simulink model "motor_supervisor"  (R2023b)
settings: Solver=FixedStepDiscrete  StartTime=0.0  StopTime=10.0  FixedStep=1e-3  RelTol=1e-3  EnableMultiTasking=on
settings Model: DataDictionary=common.sldd  Creator=mfussi  LastModifiedBy=mfussi
settings SolverCC: AutoInsertRateTranBlk=on  InsertRTBMode=Never (minimum delay)
settings DataIOCC: SaveOutput=off  SignalLogging=off  DSMLogging=off  StreamToWks=off  SaveTime=off  ReturnWorkspaceOutputs=off
settings OptimizationCC: DefaultParameterBehavior=Inlined  UseDivisionForNetSlopeComputation=on  GainParamInheritBuiltInType=on  UseFloatMulNetSlope=on  InlineInvariantSignals=on  EnhancedBackFolding=on  NoFixptDivByZeroProtection=on  EfficientFloat2IntCast=on  OptimizeBlockOrder=speed  DifferentSizesBufferReuse=on  OptimizationCustomize=off  EfficientTunableParamExpr=on
settings DebuggingCC: ParameterTunabilityLossMsg=error
settings HardwareCC: ProdBitPerPointer=32  ProdBitPerSizeT=32  ProdBitPerPtrDiffT=32  ProdLargestAtomicInteger=Long  ProdLargestAtomicFloat=Double  ProdWordSize=32  ProdLongLongMode=on  ProdHWDeviceType=ARM Compatible->ARM Cortex-M
settings SFSimCC: MATLABDynamicMemAlloc=off
settings SFSimCC: SimCustomHeaderCode=|
  | #include "rtw_enable_disable_motors.h"
  | #include "rtw_motor_config.h"
settings SFSimCC: SimUserSources=|
  | rtw_enable_disable_motors.c
  | rtw_motor_config.c
settings RTWCC: Description=Embedded Coder  SystemTargetFile=ert.tlc  GenCodeOnly=on  TemplateMakefile=ert_default_tmf  RTWUseSimCustomCode=on
settings RTWCC: CustomHeaderCode=|
  | #include "rtw_enable_disable_motors.h"
  | #include "rtw_motor_config.h"
settings RTWCC: CustomSource=|
  | rtw_enable_disable_motors.c
  | rtw_motor_config.c
settings CodeAppCC: ForceParamTrailComments=on  IgnoreCustomStorageClasses=off  OperatorAnnotations=on  SimulinkDataObjDesc=on  SFDataObjDesc=on  InsertBlockDesc=on
settings ERTTargetCC: TargetLangStandard=C99 (ISO)  CodeReplacementLibrary=ARM Cortex-M,iCubTech  GenerateSampleERTMain=on  CodeInterfacePackaging=Reusable function  InlinedParameterPlacement=NonHierarchical  RootIOFormat=Structure reference  ERTCustomFileTemplate=example_file_process.tlc

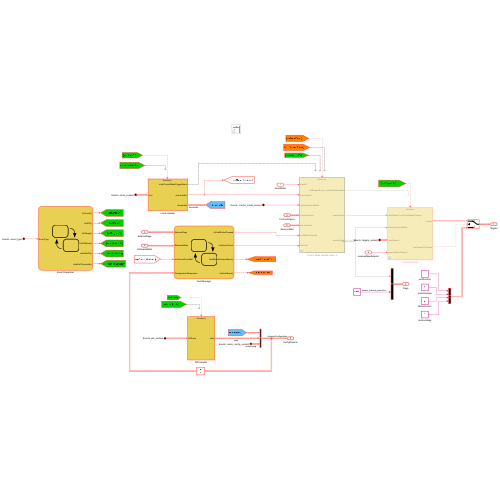
[thumbnail: Simulink's stored preview of the top-level diagram]
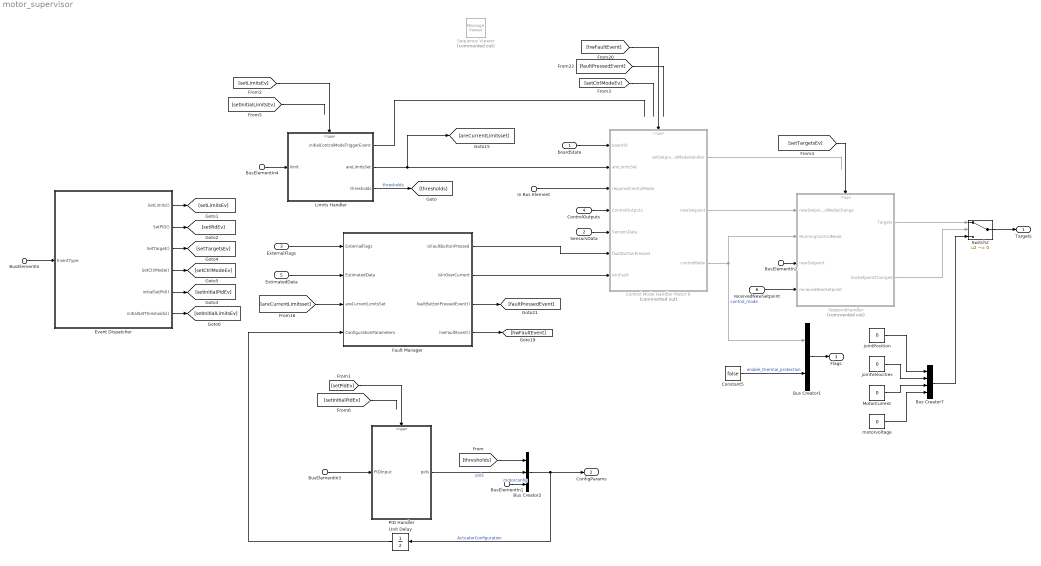
== system motor_supervisor ==
  boardState : Inport
  SensorsData : Inport  Port=2  OutDataTypeStr=Bus: SensorsData  BusOutputAsStruct=on
  ExternalFlags : Inport  Port=3  OutDataTypeStr=Bus: ExternalFlags  BusOutputAsStruct=on
  ControlOutputs : Inport  Port=4  OutDataTypeStr=Bus: FOCOutputs  BusOutputAsStruct=on
  EstimatedData : Inport  Port=5  OutDataTypeStr=Bus: EstimatedData  BusOutputAsStruct=on
  receivedNewSetpoint : Inport  Port=6
  BusElementIn2 : Inport  Port=7  PortName=Events  Element=targets_content
  BusElementIn3 : Inport  Port=7  PortName=Events  Element=pid_content
  In Bus Element : Inport  Port=7  PortName=Events  Element=control_mode_content
  BusElementIn4 : Inport  Port=7  PortName=Events  Element=limits_content
  BusElementIn : Inport  Port=7  PortName=Events  Element=event_type
  BusElementIn1 : Inport  Port=7  PortName=Events  Element=motor_config_content
  Bus Creator1 : BusCreator  Inputs=2  OutDataTypeStr=Bus: Flags  NonVirtualBus=on
      settings: InheritFromInputs=off
  Bus Creator2 : BusCreator  Inputs=3  OutDataTypeStr=Bus: ActuatorConfiguration  NonVirtualBus=on
      settings: InheritFromInputs=off
  Bus Creator7 : BusCreator  Inputs=4  OutDataTypeStr=Bus: Targets  NonVirtualBus=on
      settings: InheritFromInputs=off
  Constant5 : Constant  Value=false  OutDataTypeStr=boolean
  Control Mode Handler Motor 0 : Subsystem  Commented=on  TreatAsAtomicUnit=on
  Event Dispatcher : Stateflow chart  TreatAsAtomicUnit=on
  Fault Manager : Stateflow chart  TreatAsAtomicUnit=on
  Limits Handler : Subsystem  TreatAsAtomicUnit=on
  MotorCurrent : Constant  Value=0  OutDataTypeStr=single
  PID Handler : Subsystem
  Sequence Viewer : MessageViewer  Commented=on  History=1000  SavedRootId=#
  SetpointHandler : Subsystem  Commented=on  TreatAsAtomicUnit=on
  Switch2 : Switch  Criteria=u2 ~= 0  OutDataTypeStr=Inherit: Inherit via back propagation  SaturateOnIntegerOverflow=off  InputSameDT=off
  Unit Delay : UnitDelay  SampleTime=-1  HasFrameUpgradeWarning=on
  jointPosition : Constant  Value=0  OutDataTypeStr=single
  jointVelocities : Constant  Value=0  OutDataTypeStr=single
  motorvoltage : Constant  Value=0  OutDataTypeStr=single
  Targets : Outport  OutDataTypeStr=Bus: Targets
  ConfigParams : Outport  Port=2  OutDataTypeStr=Bus: ActuatorConfiguration
  Flags : Outport  Port=3  OutDataTypeStr=Bus: Flags
  wires:
  Switch2/1 -> Targets/1
  ControlOutputs/1 -> Control Mode Handler Motor 0/4(ControlOutputs)
  boardState/1 -> Control Mode Handler Motor 0/1(boardSt)
  ExternalFlags/1 -> Fault Manager/1(ExternalFlags)
  [setLimitsEv] -> Limits Handler/Trigger
  EstimatedData/1 -> Fault Manager/2(EstimatedData)
  [faultPressedEvent] -> ?
  Fault Manager/1(isFaultButtonPressed) -> Control Mode Handler Motor 0/6(faultButtonPressed)
  SensorsData/1 -> Control Mode Handler Motor 0/5(SensorsData)
  [setPidEv] -> PID Handler/Trigger
  Fault Manager/4(hwFaultEvent()) -> [hwFaultEvent]
  Bus Creator2/1 -> ConfigParams/1, Unit Delay/1  "ActuatorConfiguration"
  Control Mode Handler Motor 0/1(setSetpointEvent_controlModeHandler) -> ?
  Unit Delay/1 -> Fault Manager/4(ConfigurationParameters)
  MotorCurrent/1 -> Bus Creator7/3
  Fault Manager/2(isInOverCurrent) -> Control Mode Handler Motor 0/7(isInFault)
  SetpointHandler/2(hasSetpointChanged) -> Switch2/2
  In Bus Element/1 -> Control Mode Handler Motor 0/3(requiredControlMode)
  [hwFaultEvent] -> Control Mode Handler Motor 0/Trigger
  BusElementIn2/1 -> SetpointHandler/3(newSetpoint)
  BusElementIn1/1 -> Bus Creator2/3  "motorconfig"
  jointPosition/1 -> Bus Creator7/1
  [setInitialLimitsEv] -> ?
  motorvoltage/1 -> Bus Creator7/4
  SetpointHandler/1(Targets) -> Switch2/1
  BusElementIn3/1 -> PID Handler/1(PIDInput)
  [setCtrlModeEv] -> ?
  [setInitialPidEv] -> ?
  Limits Handler/2(areLimitsSet) -> Control Mode Handler Motor 0/2(areLimitsSet), [areCurrentLimitsset]
  [areCurrentLimitsset] -> Fault Manager/3(areCurrentLimitsSet)
  [thresholds] -> Bus Creator2/1
  Fault Manager/3(faultButtonPressedEvent()) -> [faultPressedEvent]
  Limits Handler/1(initialControlModeTriggerEvent) -> ?
  Limits Handler/3(thresholds) -> [thresholds]  "thresholds"
  jointVelocities/1 -> Bus Creator7/2
  Bus Creator7/1 -> Switch2/3
  BusElementIn/1 -> Event Dispatcher/1(EventType)
  Event Dispatcher/1(SetLimits()) -> [setLimitsEv]
  Event Dispatcher/2(SetPID()) -> [setPidEv]
  Event Dispatcher/3(SetTarget()) -> [setTargetsEv]
  Event Dispatcher/4(SetCtrlMode()) -> [setCtrlModeEv]
  Event Dispatcher/5(initialSetPid()) -> [setInitialPidEv]
  Event Dispatcher/6(initialSetThresholds()) -> [setInitialLimitsEv]
  Constant5/1 -> Bus Creator1/2  "enable_thermal_protection"
  Control Mode Handler Motor 0/3(controlMode) -> SetpointHandler/2(RunningControlMode), Bus Creator1/1  "control_mode"
  Bus Creator1/1 -> Flags/1
  Control Mode Handler Motor 0/2(newSetpoint) -> SetpointHandler/1(newSetpoint_onControlModeChange)
  [setTargetsEv] -> SetpointHandler/Trigger
  receivedNewSetpoint/1 -> SetpointHandler/4(receivedNewSetpoint)
  BusElementIn4/1 -> Limits Handler/1(limit)
  PID Handler/1(pids) -> Bus Creator2/2  "pids"

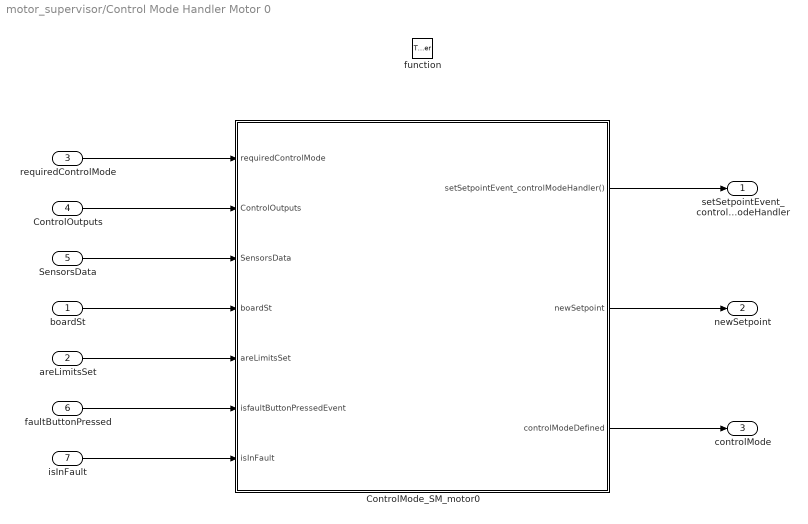
== system motor_supervisor/Control Mode Handler Motor 0 ==
  boardSt : Inport
  areLimitsSet : Inport  Port=2
  requiredControlMode : Inport  Port=3  OutDataTypeStr=Enum: ControlModes
  ControlOutputs : Inport  Port=4  OutDataTypeStr=Bus: FOCOutputs
  SensorsData : Inport  Port=5  OutDataTypeStr=Bus: SensorsData
  faultButtonPressed : Inport  Port=6  OutDataTypeStr=boolean
  isInFault : Inport  Port=7
  function : TriggerPort  TriggerType=function-call  VariantControl=(inherit)  OutputDataType=double
  ControlMode_SM_motor0 : Stateflow chart  TreatAsAtomicUnit=on
      settings: PortSchema="{\"entries\":[{\"content\":{\"sides\":[{\"content\":{\"connectorIds\":[\"In3\",\"In5\",\"In4\",\"In1\",\"In2\",\"In6\",\"In7\"]},\"type\":\"ConnectorPlacement.EquallySpacedRectSide\",\"uuid\":\"16512c25-bd76-4850-9767-5b856cef53aa\"},{\"content\":{\"connectorIds\":[\"Out3\",\"Out1\",\"Out2\"],\"side\":\"RIGHT\"},\"type\":\"ConnectorPlacement.EquallySpacedRectSide\",\"uuid\":\"18a45251-a2e9-43d4-bd88-b12ad9528921\"},{\"content\":{\"connectorIds\":[],\"side\":\"TOP\"},\"type\":\"ConnectorPlacement.EquallySpacedRectSide\",\"uuid\":\"fd5907c5-7215-4be4-b0f8-eb015da6c502\"}]},\"type\":\"ConnectorPlacement.EquallySpacedConnector\",\"uuid\":\"dd0cc5ef-a33e-40fc-9b84-b3bdf02167fe\"}],\"packageUris\":[\"http://schema.mathworks.com/mf0/Connector/R2020b\"],\"version\":\"1.0\"}"
  setSetpointEvent_controlModeHandler : Outport
  newSetpoint : Outport  Port=2  OutDataTypeStr=single
  controlMode : Outport  Port=3  OutDataTypeStr=Enum: ControlModes
  wires:
  boardSt/1 -> ControlMode_SM_motor0/1(boardSt)
  areLimitsSet/1 -> ControlMode_SM_motor0/2(areLimitsSet)
  requiredControlMode/1 -> ControlMode_SM_motor0/3(requiredControlMode)
  SensorsData/1 -> ControlMode_SM_motor0/4(SensorsData)
  ControlOutputs/1 -> ControlMode_SM_motor0/5(ControlOutputs)
  ControlMode_SM_motor0/2(controlModeDefined) -> controlMode/1
  ControlMode_SM_motor0/1(newSetpoint) -> newSetpoint/1
  ControlMode_SM_motor0/3(setSetpointEvent_controlModeHandler()) -> setSetpointEvent_controlModeHandler/1
  faultButtonPressed/1 -> ControlMode_SM_motor0/6(isfaultButtonPressedEvent)
  isInFault/1 -> ControlMode_SM_motor0/7(isInFault)

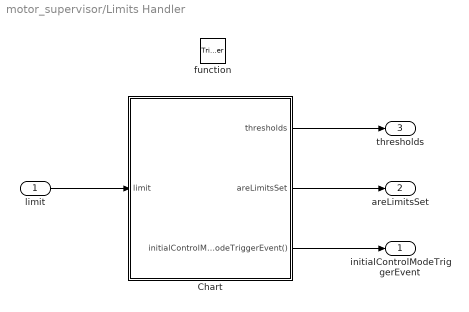
== system motor_supervisor/Limits Handler ==
  limit : Inport  OutDataTypeStr=Bus: SupervisorInputLimits
  function : TriggerPort  TriggerType=function-call  VariantControl=(inherit)
  Chart : Stateflow chart  TreatAsAtomicUnit=on
  initialControlModeTriggerEvent : Outport
  areLimitsSet : Outport  Port=2
  thresholds : Outport  Port=3
  wires:
  Chart/1(thresholds) -> thresholds/1
  Chart/2(areLimitsSet) -> areLimitsSet/1
  limit/1 -> Chart/1(limit)
  Chart/3(initialControlModeTriggerEvent()) -> initialControlModeTriggerEvent/1

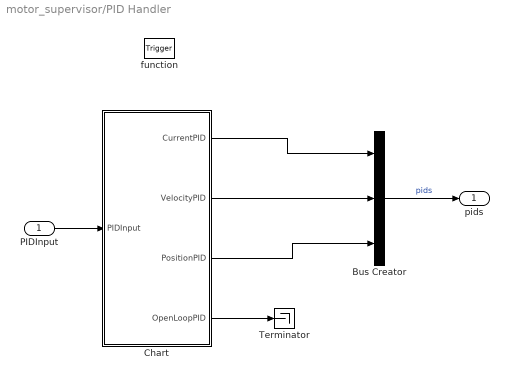
== system motor_supervisor/PID Handler ==
  PIDInput : Inport
  function : TriggerPort  TriggerType=function-call  VariantControl=(inherit)
  Bus Creator : BusCreator  Inputs=3  OutDataTypeStr=Bus: PIDsConfiguration  NonVirtualBus=on
      settings: InheritFromInputs=off
  Chart : Stateflow chart  TreatAsAtomicUnit=on
  Terminator : Terminator
  pids : Outport  OutDataTypeStr=Bus: PIDsConfiguration
  wires:
  PIDInput/1 -> Chart/1(PIDInput)
  Chart/2(VelocityPID) -> Bus Creator/2
  Chart/3(PositionPID) -> Bus Creator/3
  Chart/4(OpenLoopPID) -> Terminator/1
  Chart/1(CurrentPID) -> Bus Creator/1
  Bus Creator/1 -> pids/1  "pids"

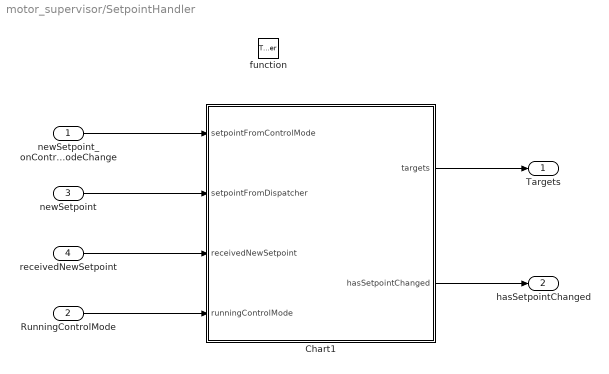
== system motor_supervisor/SetpointHandler ==
  newSetpoint_onControlModeChange : Inport
  RunningControlMode : Inport  Port=2  OutDataTypeStr=Enum: ControlModes
  newSetpoint : Inport  Port=3
  receivedNewSetpoint : Inport  Port=4
  function : TriggerPort  TriggerType=function-call  VariantControl=(inherit)
  Chart1 : Stateflow chart  TreatAsAtomicUnit=on
  Targets : Outport  OutDataTypeStr=Bus: Targets
  hasSetpointChanged : Outport  Port=2
  wires:
  newSetpoint_onControlModeChange/1 -> Chart1/1(setpointFromControlMode)
  newSetpoint/1 -> Chart1/2(setpointFromDispatcher)
  Chart1/2(hasSetpointChanged) -> hasSetpointChanged/1
  Chart1/1(targets) -> Targets/1
  receivedNewSetpoint/1 -> Chart1/3(receivedNewSetpoint)
  RunningControlMode/1 -> Chart1/4(runningControlMode)

== stateflow chart motor_supervisor/Fault Manager ==
  state FAULT_HANDLER
    state OverCurrent [parallel]
      settings: executionOrder=2
      state NoFault
        entry:
        isInOverCurrent=false;
        //MotorFaultFlags.overCurrent=0;
      note: TIP : shall we chage isConfigurationSet,
          | in one function that check only current configuration???
      state LimitNonConfigured
      state OverCurrentFault
        entry:
        //MotorFaultFlags.overCurrent=1;
        isInOverCurrent=true;
        send(hwFaultEvent);
      (default) -> LimitNonConfigured
      LimitNonConfigured -> FAULT_HANDLER.OverCurrent.NoFault : [areCurrentLimitsSet==true]
      FAULT_HANDLER.OverCurrent.NoFault -> OverCurrentFault : [abs(EstimatedData.Iq_filtered) >= ConfigurationParameters.thresholds.motorOverloadCurrents]
      OverCurrentFault -> FAULT_HANDLER.OverCurrent.NoFault : [abs(EstimatedData.Iq_filtered) < ConfigurationParameters.thresholds.motorOverloadCurrents]
    state FaultButtonPressed [parallel]
      settings: executionOrder=1
      state NoFault
        entry:
        isFaultButtonPressed = false;
      state ButtonPressed
        entry:
        isFaultButtonPressed = true;
        send(faultButtonPressedEvent);
      (default) -> FAULT_HANDLER.FaultButtonPressed.NoFault
      ButtonPressed -> FAULT_HANDLER.FaultButtonPressed.NoFault : [hasChangedTo(ExternalFlags.fault_button, false)]
      FAULT_HANDLER.FaultButtonPressed.NoFault -> ButtonPressed : [hasChangedTo(ExternalFlags.fault_button, true)]
  data: isFaultButtonPressed output boolean =false; ExternalFlags input Bus: ExternalFlags; EstimatedData input Bus: EstimatedData; areCurrentLimitsSet input boolean; isInOverCurrent output boolean =false; ConfigurationParameters input Bus: ActuatorConfiguration
  events: faultButtonPressedEvent output FUNCTION_CALL_EVENT; hwFaultEvent output FUNCTION_CALL_EVENT

== stateflow chart motor_supervisor/Event Dispatcher ==
  state Home
  (default) -> (junction 17) : {
      | //Startup Events
      | send(initialSetPid);
      | send(initialSetThresholds)
      | }
  (junction 17) -> Home
  Home -> Home [order 3] : [EventType == SupervisorEvents.SetTarget]{send(SetTarget)}
  Home -> Home [order 1] : [EventType == SupervisorEvents.SetLimit]{send(SetLimits)}
  Home -> Home [order 4] : [EventType == SupervisorEvents.SetControlMode]{send(SetCtrlMode)}
  Home -> Home [order 2] : [EventType == SupervisorEvents.SetPid]{send(SetPID)}
  data: EventType input Enum: SupervisorEvents
  events: SetLimits output FUNCTION_CALL_EVENT; SetPID output FUNCTION_CALL_EVENT; SetTarget output FUNCTION_CALL_EVENT; SetCtrlMode output FUNCTION_CALL_EVENT; initialSetPid output FUNCTION_CALL_EVENT; initialSetThresholds output FUNCTION_CALL_EVENT

== stateflow chart motor_supervisor/PID Handler/Chart ==
  state home
  (default) -> (junction 7)
  (junction 7) -> (junction 9) : {PositionPID = InitConfParams.pids.positionPID;}
  (junction 9) -> (junction 17) [order 5]
  (junction 34) -> (junction 9)
  (junction 9) -> (junction 37) [order 4] : [PIDInput.type == ControlModes.Velocity]
  (junction 9) -> (junction 15) [order 3] : [PIDInput.type == ControlModes.Voltage]
  (junction 9) -> (junction 11) [order 1] : [PIDInput.type == ControlModes.Current]
  (junction 17) -> (junction 27)
  (junction 32) -> (junction 34)
  (junction 9) -> (junction 13) [order 2] : [PIDInput.type == ControlModes.Position]
  (junction 11) -> (junction 19) : {CurrentPID.P = PIDInput.P;
      | CurrentPID.I = PIDInput.I;
      | CurrentPID.D = PIDInput.D;
      | CurrentPID.shift_factor = PIDInput.shift_factor;
      | CurrentPID.type = ControlModes.Current;}
  (junction 13) -> home : {PositionPID.P = 9;
      | PositionPID.I = 15;
      | PositionPID.D = 7;
      | PositionPID.shift_factor = PIDInput.shift_factor;
      | PositionPID.type = ControlModes.Position;}
  (junction 15) -> (junction 24) : {OpenLoopPID.P = PIDInput.P;
      | OpenLoopPID.I = PIDInput.I;
      | OpenLoopPID.D = PIDInput.D;
      | OpenLoopPID.shift_factor = PIDInput.shift_factor;}
  (junction 37) -> (junction 39) : {VelocityPID.P = PIDInput.P;
      | VelocityPID.I = PIDInput.I;
      | VelocityPID.D = PIDInput.D;
      | VelocityPID.shift_factor = PIDInput.shift_factor;}
  (junction 27) -> (junction 39)
  (junction 39) -> (junction 24)
  (junction 19) -> home
  (junction 24) -> home
  home -> (junction 30)
  (junction 30) -> (junction 32)
  data: PIDInput input Bus: PID; CurrentPID output Bus: PID; VelocityPID output Bus: PID; PositionPID output Bus: PID; OpenLoopPID output Bus: PID; InitConfParams local Bus: ActuatorConfiguration

== stateflow chart motor_supervisor/SetpointHandler/Chart1 ==
  note: The idea here is : first of all reset all the targets and then set only the value of the given setpoint. If we are in idel or HW fault all targets remain equal to 0.
  state init
  (junction 54) -> (junction 75) [order 1] : [CheckSetPointVoltage()]{newSetpoint = setpointFromDispatcher.motorvoltage;}
  (junction 75) -> (junction 77)
  (default) -> (junction 8)
  (junction 54) -> (junction 77) [order 2] : [CheckSetPointCurrent()]{newSetpoint = setpointFromDispatcher.motorcurrent;}
  (junction 77) -> (junction 79)
  (junction 8) -> (junction 54) [order 1] : [receivedNewSetpoint==true]
  (junction 9) -> (junction 8)
  (junction 54) -> (junction 79) [order 3] : [CheckSetPointVelocity()]{newSetpoint = setpointFromDispatcher.jointvelocities;}
  (junction 54) -> (junction 81) [order 4] : {newSetpoint = 0;}
  (junction 8) -> (junction 59) [order 2] : {newSetpoint=setpointFromControlMode}
  (junction 22) -> (junction 9)
  (junction 79) -> (junction 81)
  (junction 81) -> (junction 59)
  (junction 59) -> (junction 6) : {targets.motorvoltage = 0;
      | targets.motorcurrent = 0;
      | targets.jointvelocities =0;
      | targets.jointpositions = 0;}
  (junction 6) -> (junction 11) [order 5]
  (junction 6) -> (junction 28) [order 4] : [CheckSetPointPosition()]
  (junction 6) -> (junction 19) [order 2] : [CheckSetPointVoltage()]
  (junction 6) -> (junction 18) [order 3] : [CheckSetPointVelocity()]
  (junction 6) -> (junction 20) [order 1] : [CheckSetPointCurrent()]
  (junction 11) -> (junction 32)
  (junction 18) -> (junction 14) : {targets.jointvelocities = newSetpoint;}
  (junction 28) -> (junction 16) : {targets.jointpositions = newSetpoint;}
  (junction 19) -> (junction 31) : {targets.motorvoltage = newSetpoint;}
  (junction 20) -> (junction 24) : {targets.motorcurrent = newSetpoint;}
  (junction 16) -> (junction 14)
  (junction 14) -> (junction 15)
  (junction 31) -> (junction 24)
  (junction 24) -> (junction 15)
  (junction 15) -> init : {hasSetpointChanged = true;}
  init -> (junction 22)
  (junction 32) -> init
  data: out function_output boolean size=1; out function_output boolean size=1; out function_output boolean size=1; out function_output boolean size=1; setpointFromControlMode input single; setpointFromDispatcher input Bus: Targets; targets output Bus: Targets; hasSetpointChanged output boolean =false; newSetpoint local single size=1; receivedNewSetpoint input boolean; runningControlMode input Enum: ControlModes
  function out = CheckSetPointCurrent:
    | function out = CheckSetPointCurrent
    |  
    | if (runningControlMode ==ControlModes.Current )
    |     out = true;
    | else 
    |     out = false;
    | end
  function out = CheckSetPointVoltage:
    | function out = CheckSetPointVoltage
    |  
    | if (runningControlMode ==ControlModes.Voltage )
    |     out = true;
    | else 
    |     out = false;
    | end
  function out = CheckSetPointPosition:
    | function out = CheckSetPointPosition
    |  
    | if (runningControlMode ==ControlModes.Position )
    |     out = true;
    | else 
    |     out = false;
    | end
  function out = CheckSetPointVelocity:
    | function out = CheckSetPointVelocity
    |  
    | if (runningControlMode ==ControlModes.Velocity )
    |     out = true;
    | else 
    |     out = false;
    | end

== stateflow chart motor_supervisor/Control Mode Handler Motor 0/ControlMode_SM_motor0 ==
  state Torque [commented out]
  state NotConfigured
    entry:
    controlModeDefined = ControlModes.NotConfigured;
    // rtw_disableMotor();
  state Idle
    entry:
    controlModeDefined = ControlModes.Idle;
    // rtw_disableMotor();
    //rtw_enableMotor()
    //this updates the targets value
    send(setSetpointEvent_controlModeHandler);
  state Position
    entry:
    controlModeDefined = ControlModes.Position;
    newSetpoint=SensorsData.jointpositions;
    send(setSetpointEvent_controlModeHandler);
  state Current
    entry:
    controlModeDefined = ControlModes.Current;
    send(setSetpointEvent_controlModeHandler);
  state HWFault
    entry:
    controlModeDefined = ControlModes.HwFaultCM;
    // rtw_disableMotor();
    //this updates the targets value
    send(setSetpointEvent_controlModeHandler);
  state Voltage
    entry:
    controlModeDefined = ControlModes.Voltage;
    send(setSetpointEvent_controlModeHandler);
  note: IMPORTANT:
      | Currently we use IDLE command to exit from HWFault state,
      | but We should use FORCE_IDLE command when it will be implemented
  state Velocity
    entry:
    controlModeDefined = ControlModes.Velocity;
    newSetpoint=0;
    send(setSetpointEvent_controlModeHandler);
  (junction 353) -> (junction 355)
  (junction 350) -> (junction 353) [order 1] : [IsBoardReady() && isConfigurationSet()]
  (junction 355) -> (junction 214)
  (default) -> (junction 350)
  (junction 350) -> NotConfigured [order 2]
  NotConfigured -> (junction 213) [order 1] : [IsBoardReady() && isConfigurationSet()]
  (junction 213) -> (junction 214)
  (junction 211) -> (junction 214)
  (junction 329) -> (junction 213)
  (junction 214) -> Idle
  (junction 241) -> (junction 211)
  HWFault -> NotConfigured [order 1] : [!isInFault && IsNewCtrl_Idle() && !isConfigurationSet()]
  NotConfigured -> HWFault [order 2] : [isInFault]
  (junction 212) -> Idle
  (junction 220) -> (junction 212)
  Idle -> (junction 215) [order 2]
  (junction 215) -> Idle [order 2]
  (junction 215) -> (junction 221) [order 1] : [!IsNewCtrl_Idle()]
  (junction 216) -> Idle : [IsNewCtrl_Idle()]
  (junction 224) -> (junction 216) [order 2]
  (junction 217) -> Idle : [IsNewCtrl_Idle()]
  (junction 223) -> (junction 217) [order 2]
  (junction 218) -> Idle : [IsNewCtrl_Idle()]
  (junction 226) -> (junction 218) [order 2]
  Idle -> (junction 222) [order 1] : [isInFault || isfaultButtonPressedEvent]
  (junction 222) -> (junction 219)
  (junction 219) -> (junction 229)
  Position -> (junction 220) [order 3] : [IsNewCtrl_Idle()]
  (junction 221) -> Position [order 1] : [IsNewCtrl_Position()]
  (junction 221) -> (junction 227) [order 2]
  (junction 224) -> Position [order 1] : [IsNewCtrl_Position()]
  (junction 331) -> (junction 224) [order 1] : [!IsNewCtrl_Current()]
  Position -> (junction 225) [order 2] : [!IsNewCtrl_Idle()]
  (junction 225) -> (junction 332) : [!IsNewCtrl_Position()]
  (junction 223) -> Position [order 1] : [IsNewCtrl_Position()]
  (junction 335) -> (junction 223) [order 2]
  (junction 226) -> Position [order 1] : [IsNewCtrl_Position()]
  (junction 338) -> (junction 226) [order 2]
  Position -> (junction 228) [order 1] : [isInFault || isfaultButtonPressedEvent]
  (junction 228) -> (junction 229)
  (junction 229) -> (junction 330)
  (junction 227) -> Current [order 1] : [IsNewCtrl_Current()]{ newSetpoint=0; }
  (junction 331) -> Current [order 2]
  (junction 227) -> (junction 339) [order 2]
  Current -> (junction 331) [order 3]
  (junction 332) -> (junction 333) [order 1] : [IsNewCtrl_Current()]
  (junction 333) -> Current : {newSetpoint=ControlOutputs.Iq_fbk;}
  (junction 332) -> (junction 341) [order 2]
  (junction 335) -> (junction 334) [order 1] : [IsNewCtrl_Current()]
  (junction 334) -> (junction 337)
  (junction 343) -> (junction 335) [order 1] : [!IsNewCtrl_Voltage()]
  Current -> (junction 336) [order 2] : [!IsNewCtrl_Idle() && !IsNewCtrl_Position()]
  (junction 336) -> Current [order 2]
  (junction 336) -> (junction 346) [order 1] : [!IsNewCtrl_Current()]
  (junction 337) -> Current : {newSetpoint=ControlOutputs.Iq_fbk;}
  (junction 338) -> (junction 337) [order 1] : [IsNewCtrl_Current()]
  HWFault -> (junction 329) [order 2] : [!isInFault && IsNewCtrl_Idle()]
  (junction 347) -> (junction 338) [order 2]
  Current -> (junction 340) [order 1] : [isInFault || isfaultButtonPressedEvent]
  (junction 340) -> (junction 330)
  (junction 330) -> (junction 189)
  (junction 236) -> HWFault
  (junction 339) -> Voltage [order 1] : [IsNewCtrl_Voltage()]{newSetpoint=0; }
  (junction 339) -> (junction 186) [order 2]
  (junction 341) -> (junction 342) [order 1] : [IsNewCtrl_Voltage()]
  (junction 342) -> Voltage : {newSetpoint=ControlOutputs.Vq;}
  (junction 343) -> Voltage [order 2]
  (junction 341) -> (junction 184) [order 2]
  (junction 344) -> (junction 342)
  Voltage -> (junction 343) [order 3]
  (junction 346) -> (junction 344) [order 1] : [IsNewCtrl_Voltage()]
  (junction 346) -> (junction 185) [order 2]
  (junction 345) -> Voltage : {newSetpoint=ControlOutputs.Vq;}
  (junction 347) -> (junction 345) [order 1] : [IsNewCtrl_Voltage()]
  Voltage -> (junction 188) [order 2] : [IsNewCtrl_Velocity()]
  (junction 239) -> (junction 347) [order 1] : [!IsNewCtrl_Velocity()]
  (junction 188) -> Voltage [order 2]
  (junction 188) -> (junction 234) [order 1] : [!IsNewCtrl_Voltage()]
  Voltage -> (junction 187) [order 1] : [isInFault || isfaultButtonPressedEvent]
  (junction 187) -> (junction 189)
  (junction 189) -> (junction 235)
  (junction 186) -> Velocity : [IsNewCtrl_Velocity()]
  (junction 184) -> Velocity : [IsNewCtrl_Velocity()]
  (junction 185) -> Velocity : [IsNewCtrl_Velocity()]
  (junction 239) -> Velocity [order 2]
  (junction 234) -> Velocity : [IsNewCtrl_Velocity()]
  Velocity -> (junction 239) [order 2]
  Velocity -> (junction 240) [order 1] : [isInFault || isfaultButtonPressedEvent]
  (junction 240) -> (junction 235)
  (junction 235) -> (junction 237)
  (junction 237) -> (junction 241) [order 2] : [isfaultButtonPressedEvent]
  (junction 237) -> (junction 236) [order 1] : [isInFault]
  data: isSet function_output boolean; boardIsOK function_output boolean; out function_output boolean; out function_output boolean; out function_output boolean; out function_output boolean; out function_output boolean; boardSt input; areLimitsSet input; requiredControlMode input Enum: ControlModes; SensorsData input Bus: SensorsData; ControlOutputs input Bus: FOCOutputs; newSetpoint output single; controlModeDefined output Enum: ControlModes; isfaultButtonPressedEvent input boolean; isInFault input boolean
  events: setSetpointEvent_controlModeHandler output FUNCTION_CALL_EVENT
  function isSet = isConfigurationSet:
    | function isSet = isConfigurationSet
    | 
    | % TODO: Add more conditions as more CAN packets are processed.
    | isSet = areLimitsSet; % && IsVoltageLimitSet && IsTemperatureLimitSet;
    | %isSet = isSet && a;
    | end
  function boardIsOK=IsBoardReady:
    | function boardIsOK=IsBoardReady
    |  
    | boardIsOK = (boardSt==BoardState.Configured);
    | 
    | end
  function out=IsNewCtrl_Idle:
    | function out=IsNewCtrl_Idle
    | if(requiredControlMode==ControlModes.Idle)
    |     out=true;
    | else
    |     out=false;
    | end
  function out=IsNewCtrl_Position:
    | function out=IsNewCtrl_Position
    | if(requiredControlMode==ControlModes.Position) 
    |     out=true;
    | else
    |     out=false;
    | end
  function out=IsNewCtrl_Current:
    | function out=IsNewCtrl_Current
    | if(requiredControlMode==ControlModes.Current)
    |     out=true;
    | else
    |     out=false;
    | end
  function out=IsNewCtrl_Velocity:
    | function out=IsNewCtrl_Velocity
    | if(requiredControlMode==ControlModes.Velocity)
    |     out=true;
    | else
    |     out=false;
    | end
  function out=IsNewCtrl_Voltage:
    | function out=IsNewCtrl_Voltage
    | if(requiredControlMode==ControlModes.Voltage)
    |     out=true;
    | else
    |     out=false;
    | end

== stateflow chart motor_supervisor/Limits Handler/Chart ==
  state Home
  (junction 31) -> (junction 33)
  (junction 11) -> (junction 31) [order 1] : [areLimitsSet == false]
      | {areLimitsSet = true;
      | send(initialControlModeTriggerEvent);}
  (junction 33) -> (junction 21)
  (junction 11) -> (junction 21) [order 2]
  (junction 2) -> (junction 11) [order 1] : [limit.type == ControlModes.Current]
      | {thresholds.motorNominalCurrents = abs(limit.nominal);
      | thresholds.motorPeakCurrents = abs(limit.peak);
      | thresholds.motorOverloadCurrents = abs(limit.overload);}
  (junction 21) -> Home
  (default) -> (junction 2) : {thresholds=InitConfParams.thresholds;}
  Home -> (junction 2)
  (junction 2) -> (junction 16) [order 2]
  (junction 25) -> Home
  (junction 16) -> (junction 25)
  data: thresholds output Bus: Thresholds; areLimitsSet output boolean =false; limit input Bus: SupervisorInputLimits; InitConfParams local Bus: ActuatorConfiguration
  events: initialControlModeTriggerEvent output FUNCTION_CALL_EVENT
